simulink model "Nonlinear_Robust_Dr_CAN_04282018"  (R2015a)
settings: Solver=ode45  StartTime=0.0  StopTime=5  RelTol=1e-3
settings Model: Creator=tianwew  LastModifiedBy=tianwew

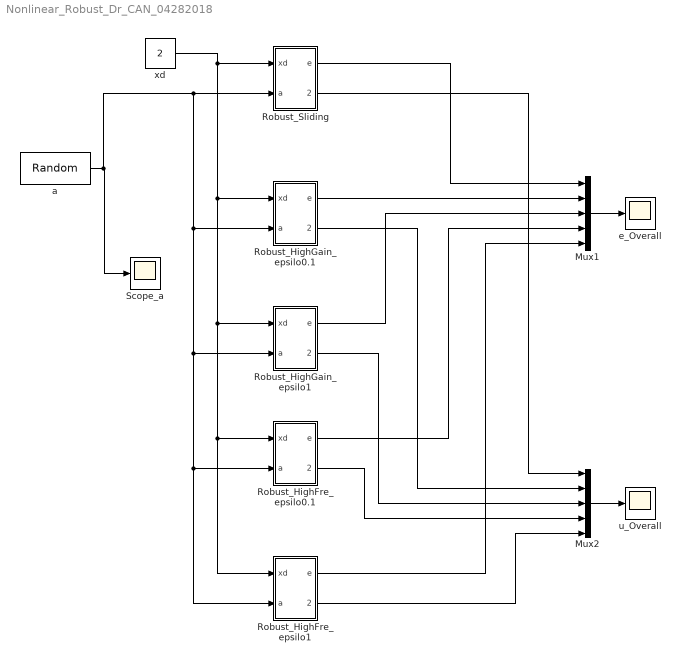
== system Nonlinear_Robust_Dr_CAN_04282018 ==
  Mux1 : Mux  Inputs=5
  Mux2 : Mux  Inputs=5
  Robust_HighFre_epsilo0.1 : Subsystem
  Robust_HighFre_epsilo1 : Subsystem
  "Robust_HighGain_epsilo0.1 " : Subsystem
  Robust_HighGain_epsilo1 : Subsystem
  "Robust_Sliding " : Subsystem
  "Scope_a " : Scope
  a : UniformRandomNumber  SampleTime=0.1
  e_Overall : Scope
      settings: ShowLegends=on  TimeRange=5  YMin=-0.5  YMax=2  SaveName=ScopeData7
  u_Overall : Scope
      settings: ShowLegends=on  SaveName=ScopeData3
  xd : Constant  Value=2
  wires:
  a/1 -> Robust_HighGain_epsilo1/2(a), Robust_HighFre_epsilo1/2(a), Robust_HighFre_epsilo0.1/2(a), "Robust_HighGain_epsilo0.1 "/2(a), "Robust_Sliding "/2(a), "Scope_a "/1
  Mux1/1 -> e_Overall/1
  xd/1 -> Robust_HighGain_epsilo1/1(xd), Robust_HighFre_epsilo1/1(xd), Robust_HighFre_epsilo0.1/1(xd), "Robust_HighGain_epsilo0.1 "/1(xd), "Robust_Sliding "/1(xd)
  "Robust_Sliding "/1(e) -> Mux1/1
  "Robust_HighGain_epsilo0.1 "/1(e) -> Mux1/2
  Robust_HighGain_epsilo1/1(e) -> Mux1/3
  Robust_HighFre_epsilo0.1/1(e) -> Mux1/4
  Robust_HighFre_epsilo1/1(e) -> Mux1/5
  Robust_HighFre_epsilo1/2("Input ") -> Mux2/5
  Robust_HighFre_epsilo0.1/2("Input ") -> Mux2/4
  Robust_HighGain_epsilo1/2("Input ") -> Mux2/3
  "Robust_HighGain_epsilo0.1 "/2("Input ") -> Mux2/2
  "Robust_Sliding "/2("Input ") -> Mux2/1
  Mux2/1 -> u_Overall/1

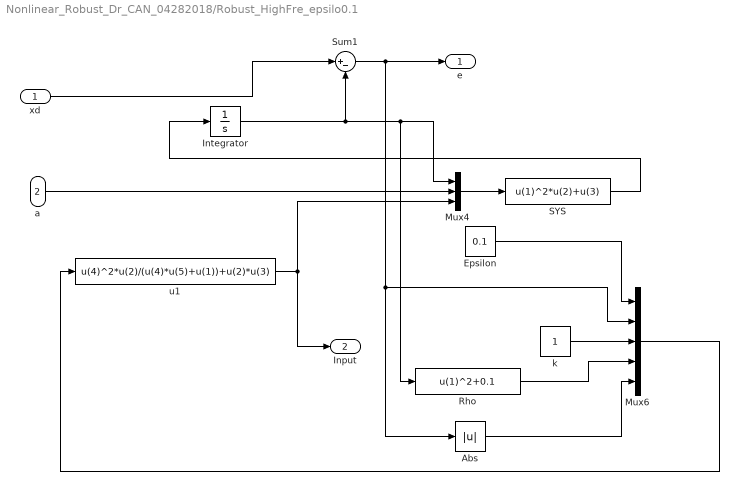
== system Nonlinear_Robust_Dr_CAN_04282018/Robust_HighFre_epsilo0.1 ==
  xd : Inport
  a : Inport  Port=2
  Abs : Abs
  Epsilon : Constant  Value=0.1
  Integrator : Integrator
  Mux4 : Mux  Inputs=3
  Mux6 : Mux  Inputs=5
  Rho : Fcn  Expr=u(1)^2+0.1
  SYS : Fcn  Expr=u(1)^2*u(2)+u(3)
  Sum1 : Sum  Inputs=|+-
  k : Constant
  u1 : Fcn  Expr=u(4)^2*u(2)/(u(4)*u(5)+u(1))+u(2)*u(3)
  e : Outport
  "Input " : Outport  Port=2
  wires:
  u1/1 -> Mux4/3, "Input "/1
  xd/1 -> Sum1/1
  Rho/1 -> Mux6/4
  Sum1/1 -> e/1, Abs/1, Mux6/2
  a/1 -> Mux4/2
  Integrator/1 -> Sum1/2, Mux4/1, Rho/1
  Mux6/1 -> u1/1
  k/1 -> Mux6/3
  SYS/1 -> Integrator/1
  Mux4/1 -> SYS/1
  Epsilon/1 -> Mux6/1
  Abs/1 -> Mux6/5

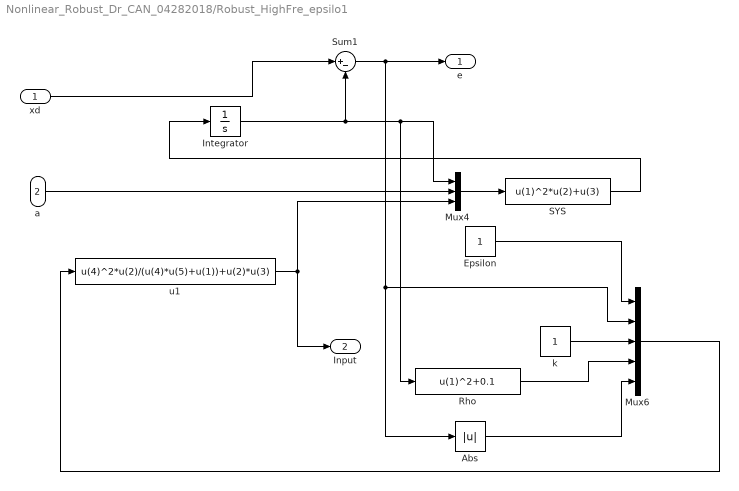
== system Nonlinear_Robust_Dr_CAN_04282018/Robust_HighFre_epsilo1 ==
  xd : Inport
  a : Inport  Port=2
  Abs : Abs
  Epsilon : Constant
  Integrator : Integrator
  Mux4 : Mux  Inputs=3
  Mux6 : Mux  Inputs=5
  Rho : Fcn  Expr=u(1)^2+0.1
  SYS : Fcn  Expr=u(1)^2*u(2)+u(3)
  Sum1 : Sum  Inputs=|+-
  k : Constant
  u1 : Fcn  Expr=u(4)^2*u(2)/(u(4)*u(5)+u(1))+u(2)*u(3)
  e : Outport
  "Input " : Outport  Port=2
  wires:
  u1/1 -> Mux4/3, "Input "/1
  xd/1 -> Sum1/1
  Rho/1 -> Mux6/4
  Sum1/1 -> e/1, Abs/1, Mux6/2
  a/1 -> Mux4/2
  Integrator/1 -> Sum1/2, Mux4/1, Rho/1
  Mux6/1 -> u1/1
  k/1 -> Mux6/3
  SYS/1 -> Integrator/1
  Mux4/1 -> SYS/1
  Epsilon/1 -> Mux6/1
  Abs/1 -> Mux6/5

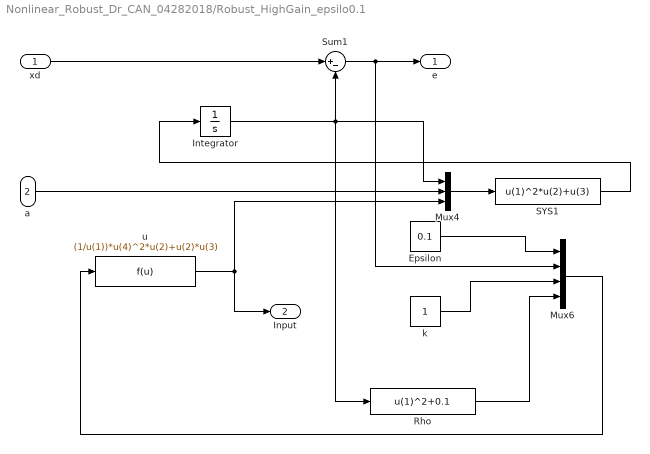
== system Nonlinear_Robust_Dr_CAN_04282018/Robust_HighGain_epsilo0.1  ==
  xd : Inport
  a : Inport  Port=2
  Epsilon : Constant  Value=0.1
  Integrator : Integrator
  Mux4 : Mux  Inputs=3
  Mux6 : Mux
  Rho : Fcn  Expr=u(1)^2+0.1
  SYS1 : Fcn  Expr=u(1)^2*u(2)+u(3)
  Sum1 : Sum  Inputs=|+-
  k : Constant
  u : Fcn  Expr=(1/u(1))*u(4)^2*u(2)+u(2)*u(3)
  e : Outport
  "Input " : Outport  Port=2
  wires:
  u/1 -> "Input "/1, Mux4/3
  xd/1 -> Sum1/1
  Rho/1 -> Mux6/4
  Sum1/1 -> Mux6/2, e/1
  a/1 -> Mux4/2
  Integrator/1 -> Mux4/1, Rho/1, Sum1/2
  Mux6/1 -> u/1
  k/1 -> Mux6/3
  SYS1/1 -> Integrator/1
  Mux4/1 -> SYS1/1
  Epsilon/1 -> Mux6/1

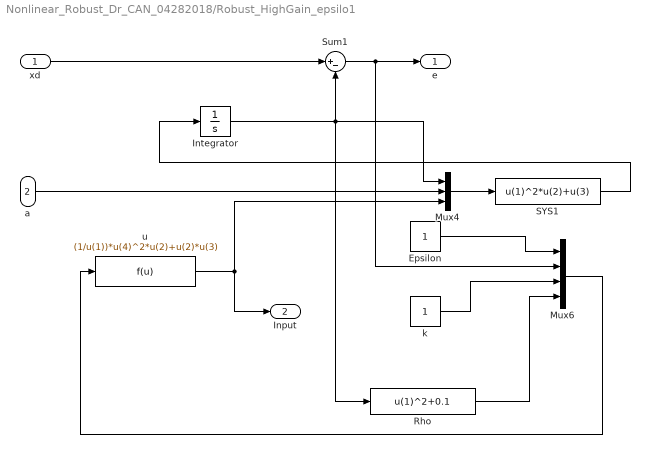
== system Nonlinear_Robust_Dr_CAN_04282018/Robust_HighGain_epsilo1 ==
  xd : Inport
  a : Inport  Port=2
  Epsilon : Constant
  Integrator : Integrator
  Mux4 : Mux  Inputs=3
  Mux6 : Mux
  Rho : Fcn  Expr=u(1)^2+0.1
  SYS1 : Fcn  Expr=u(1)^2*u(2)+u(3)
  Sum1 : Sum  Inputs=|+-
  k : Constant
  u : Fcn  Expr=(1/u(1))*u(4)^2*u(2)+u(2)*u(3)
  e : Outport
  "Input " : Outport  Port=2
  wires:
  u/1 -> "Input "/1, Mux4/3
  xd/1 -> Sum1/1
  Rho/1 -> Mux6/4
  Sum1/1 -> Mux6/2, e/1
  a/1 -> Mux4/2
  Integrator/1 -> Mux4/1, Rho/1, Sum1/2
  Mux6/1 -> u/1
  k/1 -> Mux6/3
  SYS1/1 -> Integrator/1
  Mux4/1 -> SYS1/1
  Epsilon/1 -> Mux6/1

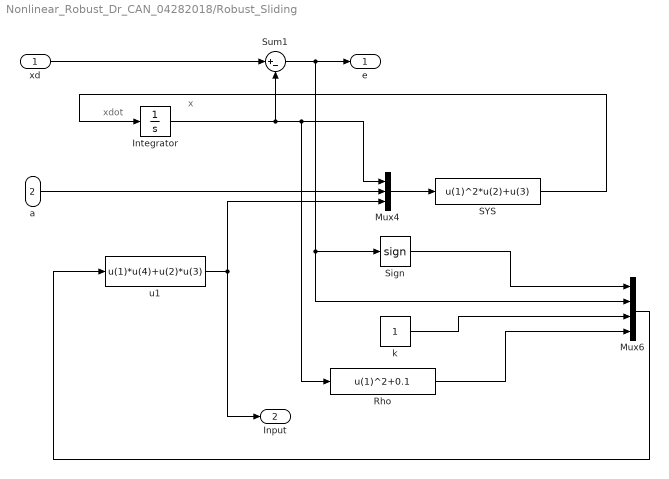
== system Nonlinear_Robust_Dr_CAN_04282018/Robust_Sliding  ==
  note: xdot
  note: x
  xd : Inport
  a : Inport  Port=2
  Integrator : Integrator
  Mux4 : Mux  Inputs=3
  Mux6 : Mux
  Rho : Fcn  Expr=u(1)^2+0.1
  SYS : Fcn  Expr=u(1)^2*u(2)+u(3)
  Sign : Signum  ZeroCross=off
  Sum1 : Sum  Inputs=|+-
  k : Constant
  u1 : Fcn  Expr=u(1)*u(4)+u(2)*u(3)
  e : Outport
  "Input " : Outport  Port=2
  wires:
  Mux4/1 -> SYS/1
  SYS/1 -> Integrator/1
  k/1 -> Mux6/3
  Mux6/1 -> u1/1
  Integrator/1 -> Mux4/1, Rho/1, Sum1/2
  a/1 -> Mux4/2
  Sum1/1 -> Mux6/2, Sign/1, e/1
  Sign/1 -> Mux6/1
  Rho/1 -> Mux6/4
  xd/1 -> Sum1/1
  u1/1 -> "Input "/1, Mux4/3
